simulink model "uncontrolled"  (R2020b)
settings: Solver=ode15s  StartTime=0  StopTime=5792.3373  MaxStep=0.1  RelTol=1e-8  AbsTol=1e-8
values from neighbouring files (symbols this model uses):
  data = struct()    [config.m]    (also in config6U.m; configSlew.m; mainOffNominal.m = dataFix)
libraries: simulink_extras x1
settings Model: SimulationMode=accelerator  Creator=pacif  LastModifiedBy=pacif

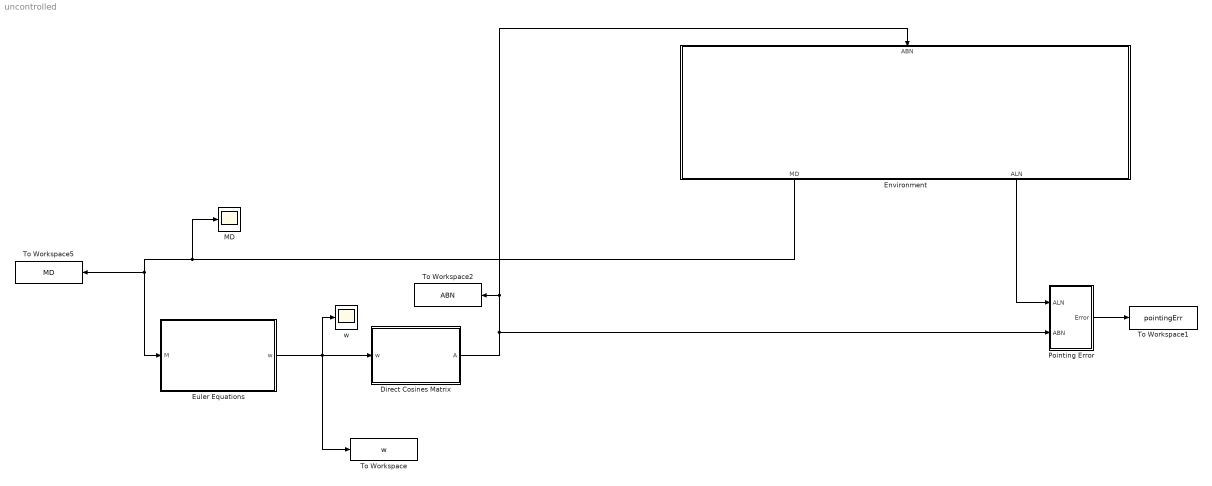
== system uncontrolled ==
  Direct Cosines Matrix : Subsystem
  Environment : Subsystem
  Euler Equations : Subsystem
  MD : Scope
  Pointing Error : Subsystem
  To Workspace : ToWorkspace  VariableName=w  SaveFormat=Timeseries  SampleTime=-1
  To Workspace1 : ToWorkspace  VariableName=pointingErr  SaveFormat=Timeseries  SampleTime=-1
  To Workspace2 : ToWorkspace  VariableName=ABN  SaveFormat=Timeseries  SampleTime=-1
  To Workspace5 : ToWorkspace  VariableName=MD  SaveFormat=Timeseries  SampleTime=-1
  w : Scope
  wires:
  Environment/1(MD) -> MD/1, To Workspace5/1, Euler Equations/1(M)
  Euler Equations/1(w) -> To Workspace/1, Direct Cosines Matrix/1(w), w/1
  Direct Cosines Matrix/1(A) -> To Workspace2/1, Environment/1(ABN), Pointing Error/2(ABN)
  Environment/2(ALN) -> Pointing Error/1(ALN)
  Pointing Error/1(Error) -> To Workspace1/1

== system uncontrolled/Direct Cosines Matrix ==
  w : Inport
  Build 3x3 Matrix : Subsystem
  Constant1 : Constant  Value=0
  Demux1 : Demux  Outputs=3
  Gain{3,5..7} (4 alike) : Gain  Gain=-1
  Integrator : Integrator  InitialCondition=data.ic.dcm
  Orthonormalization : Subsystem
  Product : Product  Multiplication=Matrix(*)
  A : Outport
  wires:
  Demux1/1 -> Build 3x3 Matrix/6(A32), Gain7/1
  Gain5/1 -> Build 3x3 Matrix/4(A12)
  Demux1/3 -> Build 3x3 Matrix/2(A21), Gain5/1
  Product/1 -> Gain3/1
  Build 3x3 Matrix/1(A) -> Product/1  "[w]^"
  Gain6/1 -> Build 3x3 Matrix/3(A31)
  Demux1/2 -> Build 3x3 Matrix/7("A13 "), Gain6/1
  Gain7/1 -> Build 3x3 Matrix/8(A23)
  Orthonormalization/1(A) -> Product/2, A/1
  Gain3/1 -> Integrator/1  "dA/dt"
  w/1 -> Demux1/1
  Integrator/1 -> Orthonormalization/1(A0)  "A"
  Constant1/1 -> Build 3x3 Matrix/1(A11), Build 3x3 Matrix/9(A33), Build 3x3 Matrix/5(A22)

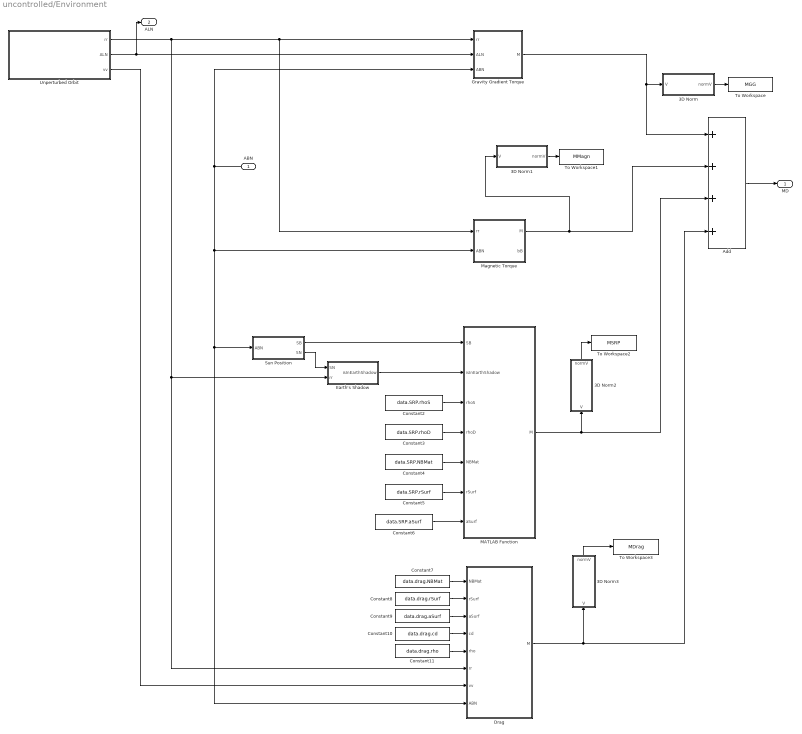
== system uncontrolled/Environment ==
  ABN : Inport
  3D Norm : Subsystem
  3D Norm1 : Subsystem
  3D Norm2 : Subsystem
  3D Norm3 : Subsystem
  Add : Sum  Inputs=++++
  Constant10 : Constant  Value=data.drag.cd
  Constant11 : Constant  Value=data.drag.rho
  Constant2 : Constant  Value=data.SRP.rhoS
  Constant3 : Constant  Value=data.SRP.rhoD
  Constant4 : Constant  Value=data.SRP.NBMat
  Constant5 : Constant  Value=data.SRP.rSurf
  Constant6 : Constant  Value=data.SRP.aSurf
  Constant7 : Constant  Value=data.drag.NBMat
  Constant8 : Constant  Value=data.drag.rSurf
  Constant9 : Constant  Value=data.drag.aSurf
  Drag : MATLAB Function  TreatAsAtomicUnit=on
  Earth's Shadow : Subsystem
  Gravity Gradient Torque : Subsystem
  MATLAB Function : MATLAB Function  TreatAsAtomicUnit=on
  Magnetic Torque : Subsystem
  "Sun Position " : Subsystem
  To Workspace : ToWorkspace  VariableName=MGG  SaveFormat=Timeseries  SampleTime=-1
  To Workspace1 : ToWorkspace  VariableName=MMagn  SaveFormat=Timeseries  SampleTime=-1
  To Workspace2 : ToWorkspace  VariableName=MSRP  SaveFormat=Timeseries  SampleTime=-1
  To Workspace3 : ToWorkspace  VariableName=MDrag  SaveFormat=Timeseries  SampleTime=-1
  Unperturbed Orbit : Subsystem
  MD : Outport
  ALN : Outport  Port=2
  wires:
  Earth's Shadow/1(isInEarthShadow) -> MATLAB Function/2(isInEarthShadow)
  Constant5/1 -> MATLAB Function/6(rSurf)
  Constant6/1 -> MATLAB Function/7(aSurf)
  Constant3/1 -> MATLAB Function/4(rhoD)
  Constant4/1 -> MATLAB Function/5(NBMat)
  Gravity Gradient Torque/1(M) -> 3D Norm/1(V), Add/1
  Unperturbed Orbit/1(rr) -> Earth's Shadow/2(rr), Drag/6(rr), Magnetic Torque/1(rr), Gravity Gradient Torque/1(rr)
  Constant10/1 -> Drag/4(cd)
  Drag/1(M) -> Add/4, 3D Norm3/1(V)
  ABN/1 -> Gravity Gradient Torque/3(ABN), Magnetic Torque/2(ABN), Drag/8(ABN), "Sun Position "/1(ABN)
  Constant7/1 -> Drag/1(NBMat)
  Constant8/1 -> Drag/2(rSurf)
  Constant9/1 -> Drag/3(aSurf)
  Add/1 -> MD/1
  Constant2/1 -> MATLAB Function/3(rhoS)
  Magnetic Torque/1(M) -> 3D Norm1/1(V), Add/2
  Unperturbed Orbit/2(ALN) -> ALN/1, Gravity Gradient Torque/2(ALN)
  Constant11/1 -> Drag/5(rho)
  Unperturbed Orbit/3(vv) -> Drag/7(vv)
  "Sun Position "/2(SN) -> Earth's Shadow/1(SN)
  "Sun Position "/1(SB) -> MATLAB Function/1(SB)
  MATLAB Function/1(M) -> Add/3, 3D Norm2/1(V)
  3D Norm/1(normV) -> To Workspace/1
  3D Norm1/1(normV) -> To Workspace1/1
  3D Norm2/1(normV) -> To Workspace2/1
  3D Norm3/1(normV) -> To Workspace3/1

== system uncontrolled/Euler Equations ==
  M : Inport
  Add : Sum
  Cross Product : Subsystem
  Gain : Gain  Gain=data.sc.invI  Multiplication=Matrix(K*u) (u vector)
  Gain2 : Gain  Gain=data.sc.inertiaMatrix  Multiplication=Matrix(K*u) (u vector)
  Integrator : Integrator  InitialCondition=data.ic.w
  w : Outport
  wires:
  Gain2/1 -> Cross Product/1(a)  "I*w"
  Cross Product/1(c) -> Add/2  "I*w x w = -w x I*w"
  M/1 -> Add/1
  Integrator/1 -> Cross Product/2(b), Gain2/1, w/1  "w"
  Gain/1 -> Integrator/1  "dw"
  Add/1 -> Gain/1

== system uncontrolled/Pointing Error ==
  ALN : Inport
  ABN : Inport  Port=2
  Acos : Trigonometry  Operator=acos
  Product : Product  Multiplication=Matrix(*)
  Radians to Degrees : simulink_extras/Transformations/Radians to Degrees
  Selector : Selector  NumberOfDimensions=2  InputPortWidth=3  IndexOptions=Index vector (dialog),Index vector (dialog)  Indices=1,1  OutputSizes=1,1
  Transpose : Math  Operator=transpose  SaturateOnIntegerOverflow=on
  Error : Outport
  wires:
  Radians to Degrees/1 -> Error/1
  ABN/1 -> Product/1
  ALN/1 -> Transpose/1
  Transpose/1 -> Product/2
  Product/1 -> Selector/1
  Selector/1 -> Acos/1
  Acos/1 -> Radians to Degrees/1

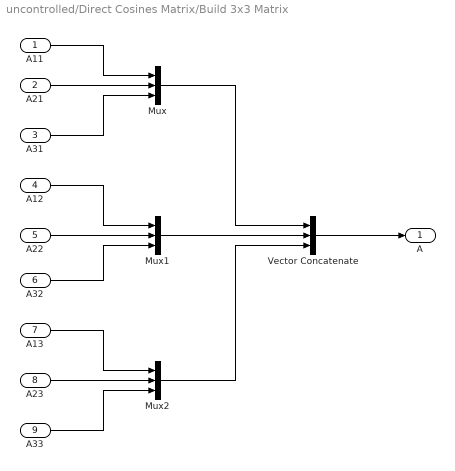
== system uncontrolled/Direct Cosines Matrix/Build 3x3 Matrix ==
  A11 : Inport
  A21 : Inport  Port=2
  A31 : Inport  Port=3
  A12 : Inport  Port=4
  A22 : Inport  Port=5
  A32 : Inport  Port=6
  "A13 " : Inport  Port=7
  A23 : Inport  Port=8
  A33 : Inport  Port=9
  Mux : Mux  Inputs=3
  Mux1 : Mux  Inputs=3
  Mux2 : Mux  Inputs=3
  Vector Concatenate : Concatenate  NumInputs=3  Mode=Multidimensional array  ConcatenateDimension=2
  A : Outport
  wires:
  A21/1 -> Mux/2
  A23/1 -> Mux2/2
  "A13 "/1 -> Mux2/1
  A11/1 -> Mux/1
  Vector Concatenate/1 -> A/1
  A31/1 -> Mux/3
  A12/1 -> Mux1/1
  A22/1 -> Mux1/2
  Mux2/1 -> Vector Concatenate/3
  Mux1/1 -> Vector Concatenate/2
  Mux/1 -> Vector Concatenate/1
  A33/1 -> Mux2/3
  A32/1 -> Mux1/3

== system uncontrolled/Direct Cosines Matrix/Orthonormalization ==
  A0 : Inport
  Add : Sum  Inputs=+-
  Gain : Gain  Gain=1.5
  Gain1 : Gain  Gain=0.5
  Product : Product  Inputs=3  Multiplication=Matrix(*)
  Transpose : Math  Operator=transpose  SaturateOnIntegerOverflow=on
  A : Outport
  wires:
  Add/1 -> A/1
  A0/1 -> Product/3, Transpose/1, Product/1, Gain/1
  Gain1/1 -> Add/2
  Gain/1 -> Add/1
  Transpose/1 -> Product/2
  Product/1 -> Gain1/1

== system uncontrolled/Environment/3D Norm ==
  V : Inport
  Add : Sum  Inputs=+++
  Demux : Demux  Outputs=3
  Square : Math  Operator=square  SaturateOnIntegerOverflow=on
  Square Root : Sqrt  SaturateOnIntegerOverflow=on
  Square1 : Math  Operator=square  SaturateOnIntegerOverflow=on
  Square2 : Math  Operator=square  SaturateOnIntegerOverflow=on
  normV : Outport
  wires:
  Square Root/1 -> normV/1
  V/1 -> Demux/1
  Demux/3 -> Square2/1
  Square/1 -> Add/1
  Demux/1 -> Square/1
  Demux/2 -> Square1/1
  Square2/1 -> Add/3
  Square1/1 -> Add/2
  Add/1 -> Square Root/1

== system uncontrolled/Environment/3D Norm1 ==
  V : Inport
  Add : Sum  Inputs=+++
  Demux : Demux  Outputs=3
  Square : Math  Operator=square  SaturateOnIntegerOverflow=on
  Square Root : Sqrt  SaturateOnIntegerOverflow=on
  Square1 : Math  Operator=square  SaturateOnIntegerOverflow=on
  Square2 : Math  Operator=square  SaturateOnIntegerOverflow=on
  normV : Outport
  wires:
  Square Root/1 -> normV/1
  V/1 -> Demux/1
  Demux/3 -> Square2/1
  Square/1 -> Add/1
  Demux/1 -> Square/1
  Demux/2 -> Square1/1
  Square2/1 -> Add/3
  Square1/1 -> Add/2
  Add/1 -> Square Root/1

== system uncontrolled/Environment/3D Norm2 ==
  V : Inport
  Add : Sum  Inputs=+++
  Demux : Demux  Outputs=3
  Square : Math  Operator=square  SaturateOnIntegerOverflow=on
  Square Root : Sqrt  SaturateOnIntegerOverflow=on
  Square1 : Math  Operator=square  SaturateOnIntegerOverflow=on
  Square2 : Math  Operator=square  SaturateOnIntegerOverflow=on
  normV : Outport
  wires:
  Square Root/1 -> normV/1
  V/1 -> Demux/1
  Demux/3 -> Square2/1
  Square/1 -> Add/1
  Demux/1 -> Square/1
  Demux/2 -> Square1/1
  Square2/1 -> Add/3
  Square1/1 -> Add/2
  Add/1 -> Square Root/1

== system uncontrolled/Environment/3D Norm3 ==
  V : Inport
  Add : Sum  Inputs=+++
  Demux : Demux  Outputs=3
  Square : Math  Operator=square  SaturateOnIntegerOverflow=on
  Square Root : Sqrt  SaturateOnIntegerOverflow=on
  Square1 : Math  Operator=square  SaturateOnIntegerOverflow=on
  Square2 : Math  Operator=square  SaturateOnIntegerOverflow=on
  normV : Outport
  wires:
  Square Root/1 -> normV/1
  V/1 -> Demux/1
  Demux/3 -> Square2/1
  Square/1 -> Add/1
  Demux/1 -> Square/1
  Demux/2 -> Square1/1
  Square2/1 -> Add/3
  Square1/1 -> Add/2
  Add/1 -> Square Root/1

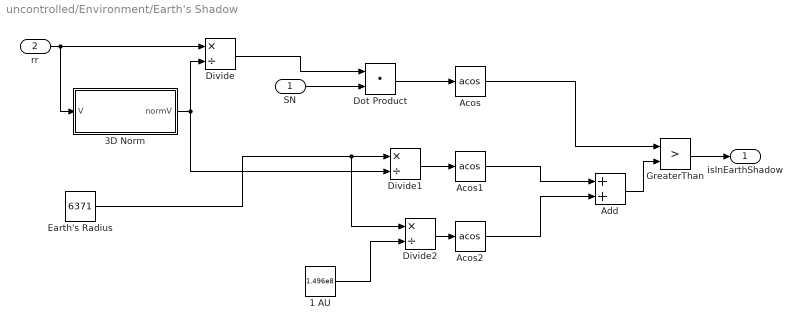
== system uncontrolled/Environment/Earth's Shadow ==
  SN : Inport
  rr : Inport  Port=2
  1 AU : Constant  Value=1.496e8
  3D Norm : Subsystem
  Acos : Trigonometry  Operator=acos
  Acos1 : Trigonometry  Operator=acos
  Acos2 : Trigonometry  Operator=acos
  Add : Sum
  Divide : Product  Inputs=*/
  Divide1 : Product  Inputs=*/
  Divide2 : Product  Inputs=*/
  Dot Product : DotProduct  InputSameDT=on  OutDataTypeStr=Inherit: Inherit via internal rule
  Earth's Radius : Constant  Value=6371
  GreaterThan : RelationalOperator  Operator=>  OutDataTypeStr=boolean  RndMeth=Simplest
  isInEarthShadow : Outport
  wires:
  SN/1 -> Dot Product/2
  GreaterThan/1 -> isInEarthShadow/1
  Add/1 -> GreaterThan/2
  Acos/1 -> GreaterThan/1
  Acos2/1 -> Add/2
  Acos1/1 -> Add/1
  rr/1 -> 3D Norm/1(V), Divide/1
  3D Norm/1(normV) -> Divide1/2, Divide/2
  Divide/1 -> Dot Product/1
  Dot Product/1 -> Acos/1
  Earth's Radius/1 -> Divide1/1, Divide2/1
  Divide1/1 -> Acos1/1
  Divide2/1 -> Acos2/1
  1 AU/1 -> Divide2/2

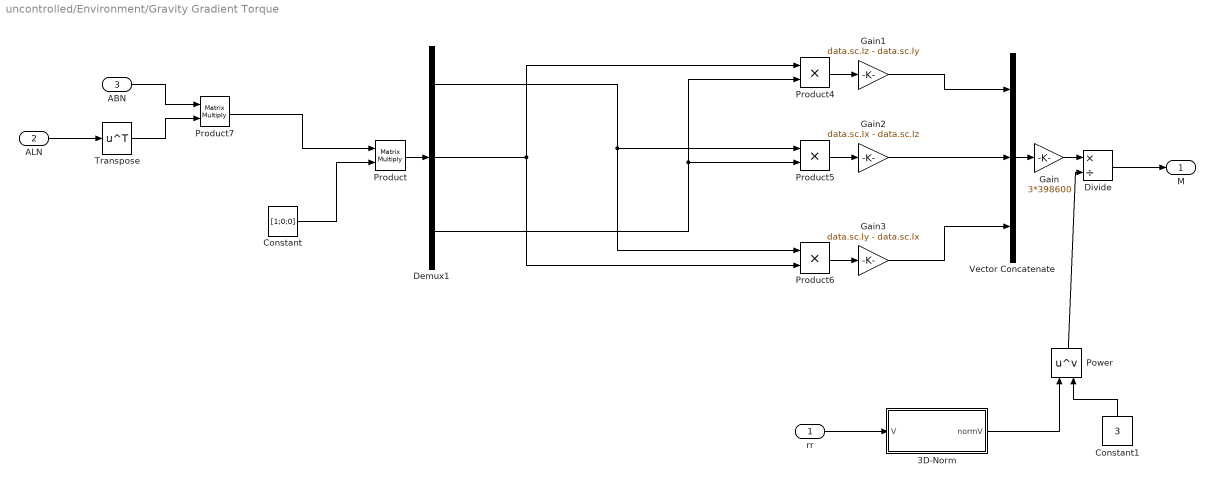
== system uncontrolled/Environment/Gravity Gradient Torque ==
  rr : Inport
  ALN : Inport  Port=2
  ABN : Inport  Port=3
  3D-Norm : Subsystem
  Constant : Constant  Value=[1;0;0]  VectorParams1D=off
  Constant1 : Constant  Value=3
  Demux1 : Demux  Outputs=3
  Divide : Product  Inputs=*/
  Gain : Gain  Gain=3*398600
  Gain1 : Gain  Gain=data.sc.Iz - data.sc.Iy
  Gain2 : Gain  Gain=data.sc.Ix - data.sc.Iz
  Gain3 : Gain  Gain=data.sc.Iy - data.sc.Ix
  Power : Math  Operator=pow  SaturateOnIntegerOverflow=on
  Product : Product  Multiplication=Matrix(*)
  Product4 : Product
  Product5 : Product
  Product6 : Product
  Product7 : Product  Multiplication=Matrix(*)
  Transpose : Math  Operator=transpose  SaturateOnIntegerOverflow=on
  Vector Concatenate : Concatenate  NumInputs=3
  M : Outport
  wires:
  Constant/1 -> Product/2
  Gain3/1 -> Vector Concatenate/3
  Gain1/1 -> Vector Concatenate/1
  Gain2/1 -> Vector Concatenate/2
  Vector Concatenate/1 -> Gain/1
  Constant1/1 -> Power/2
  Power/1 -> Divide/2
  Gain/1 -> Divide/1
  Product/1 -> Demux1/1
  Product4/1 -> Gain1/1
  Product5/1 -> Gain2/1
  Product6/1 -> Gain3/1
  Demux1/1 -> Product6/1, Product5/1
  Demux1/2 -> Product6/2, Product4/1
  Demux1/3 -> Product5/2, Product4/2
  Divide/1 -> M/1
  rr/1 -> 3D-Norm/1(V)
  3D-Norm/1(normV) -> Power/1
  ALN/1 -> Transpose/1
  Product7/1 -> Product/1
  ABN/1 -> Product7/1
  Transpose/1 -> Product7/2

== system uncontrolled/Environment/Magnetic Torque ==
  rr : Inport
  ABN : Inport  Port=2
  Cross Product : Subsystem
  Product : Product  Multiplication=Matrix(*)
  Subsystem : Subsystem
  m : Constant  Value=data.magneticTorque.m
  M : Outport
  bB : Outport  Port=2
  wires:
  rr/1 -> Subsystem/1(rr)
  ABN/1 -> Product/1
  Subsystem/1(bN) -> Product/2
  m/1 -> Cross Product/1(a)
  Product/1 -> Cross Product/2(b), bB/1
  Cross Product/1(c) -> M/1

== system uncontrolled/Environment/Sun Position  ==
  ABN : Inport
  Clock : Clock
  Cos : Trigonometry  Operator=cos
  Gain1 : Gain  Gain=2*pi/365/24/3600
  Gain2 : Gain  Gain=cos(23.45*pi/180)
  Gain3 : Gain  Gain=sin(23.45*pi/180)
  Mux : Mux  Inputs=3
  Product : Product  Multiplication=Matrix(*)
  Sin : Trigonometry
  Sin1 : Trigonometry
  SB : Outport
  SN : Outport  Port=2
  wires:
  Clock/1 -> Gain1/1
  Mux/1 -> SN/1, Product/2  "SN"
  Gain2/1 -> Mux/2
  Gain3/1 -> Mux/3
  Cos/1 -> Mux/1
  Sin1/1 -> Gain3/1
  Sin/1 -> Gain2/1
  Gain1/1 -> Sin/1, Sin1/1, Cos/1
  ABN/1 -> Product/1
  Product/1 -> SB/1

== system uncontrolled/Environment/Unperturbed Orbit ==
  Integrator : Integrator  InitialCondition=data.ic.th
  Subsystem : Subsystem
  Subsystem1 : Subsystem
  Subsystem2 : Subsystem
  Subsystem3 : Subsystem
  To Workspace : ToWorkspace  VariableName=theta  SaveFormat=Timeseries  SampleTime=-1
  rr : Outport
  ALN : Outport  Port=2
  vv : Outport  Port=3
  wires:
  Integrator/1 -> Subsystem2/1(theta), Subsystem1/1(theta), Subsystem3/1(theta), To Workspace/1, Subsystem/1(theta)
  Subsystem1/1(ALN) -> ALN/1
  Subsystem2/1(rr) -> rr/1
  Subsystem3/1(vv) -> vv/1
  Subsystem/1(theta_dot) -> Integrator/1

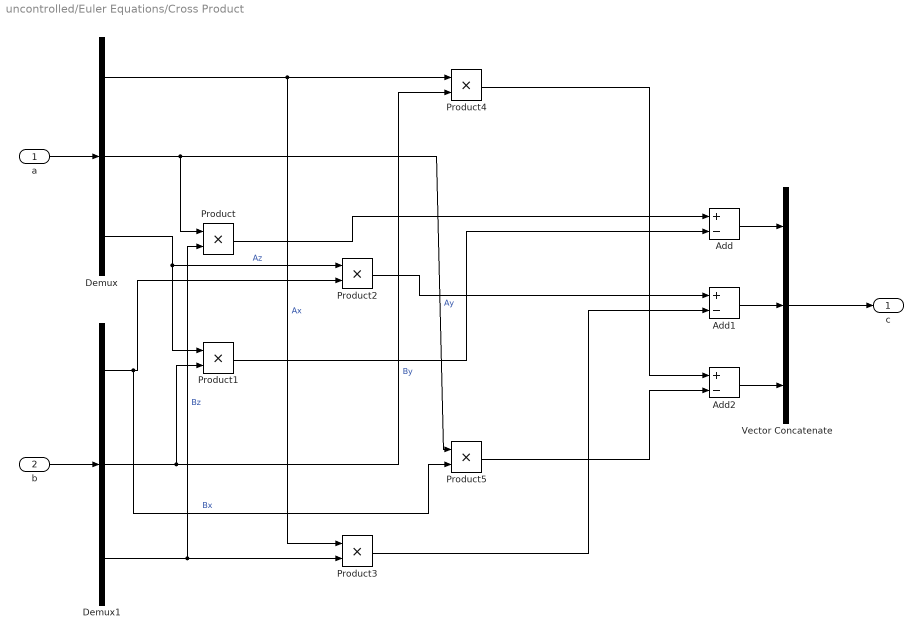
== system uncontrolled/Euler Equations/Cross Product ==
  a : Inport
  b : Inport  Port=2
  Add : Sum  Inputs=+-
  Add1 : Sum  Inputs=+-
  Add2 : Sum  Inputs=+-
  Demux : Demux  Outputs=3
  Demux1 : Demux  Outputs=3
  Product{,1..5} (6 alike) : Product
  Vector Concatenate : Concatenate  NumInputs=3
  c : Outport
  wires:
  Demux1/1 -> Product2/2, Product5/2  "Bx"
  Product2/1 -> Add1/1
  Vector Concatenate/1 -> c/1
  Add/1 -> Vector Concatenate/1
  Product3/1 -> Add1/2
  Product1/1 -> Add/2
  Product4/1 -> Add2/1
  Product/1 -> Add/1
  Demux/1 -> Product3/1, Product4/1  "Ax"
  Product5/1 -> Add2/2
  Demux/3 -> Product2/1, Product1/1  "Az"
  b/1 -> Demux1/1
  a/1 -> Demux/1
  Add2/1 -> Vector Concatenate/3
  Demux/2 -> Product5/1, Product/1  "Ay"
  Demux1/3 -> Product/2, Product3/2  "Bz"
  Demux1/2 -> Product4/2, Product1/2  "By"
  Add1/1 -> Vector Concatenate/2

== system uncontrolled/Environment/Earth's Shadow/3D Norm ==
  V : Inport
  Add : Sum  Inputs=+++
  Demux : Demux  Outputs=3
  Square : Math  Operator=square  SaturateOnIntegerOverflow=on
  Square Root : Sqrt  SaturateOnIntegerOverflow=on
  Square1 : Math  Operator=square  SaturateOnIntegerOverflow=on
  Square2 : Math  Operator=square  SaturateOnIntegerOverflow=on
  normV : Outport
  wires:
  Square Root/1 -> normV/1
  V/1 -> Demux/1
  Demux/3 -> Square2/1
  Square/1 -> Add/1
  Demux/1 -> Square/1
  Demux/2 -> Square1/1
  Square2/1 -> Add/3
  Square1/1 -> Add/2
  Add/1 -> Square Root/1

== system uncontrolled/Environment/Gravity Gradient Torque/3D-Norm ==
  V : Inport
  Add : Sum  Inputs=+++
  Demux : Demux  Outputs=3
  Square : Math  Operator=square  SaturateOnIntegerOverflow=on
  Square Root : Sqrt  SaturateOnIntegerOverflow=on
  Square1 : Math  Operator=square  SaturateOnIntegerOverflow=on
  Square2 : Math  Operator=square  SaturateOnIntegerOverflow=on
  normV : Outport
  wires:
  Square Root/1 -> normV/1
  Add/1 -> Square Root/1
  Square2/1 -> Add/3
  Square1/1 -> Add/2
  Square/1 -> Add/1
  Demux/1 -> Square/1
  Demux/2 -> Square1/1
  Demux/3 -> Square2/1
  V/1 -> Demux/1

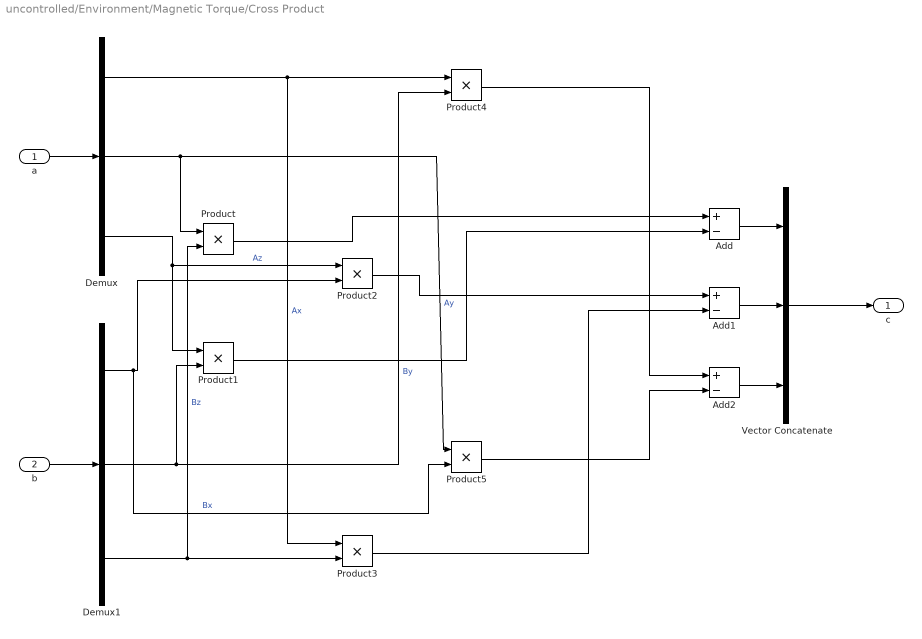
== system uncontrolled/Environment/Magnetic Torque/Cross Product ==
  a : Inport
  b : Inport  Port=2
  Add : Sum  Inputs=+-
  Add1 : Sum  Inputs=+-
  Add2 : Sum  Inputs=+-
  Demux : Demux  Outputs=3
  Demux1 : Demux  Outputs=3
  Product{,1..5} (6 alike) : Product
  Vector Concatenate : Concatenate  NumInputs=3
  c : Outport
  wires:
  Demux1/1 -> Product2/2, Product5/2  "Bx"
  Product2/1 -> Add1/1
  Vector Concatenate/1 -> c/1
  Add/1 -> Vector Concatenate/1
  Product3/1 -> Add1/2
  Product1/1 -> Add/2
  Product4/1 -> Add2/1
  Product/1 -> Add/1
  Demux/1 -> Product3/1, Product4/1  "Ax"
  Product5/1 -> Add2/2
  Demux/3 -> Product2/1, Product1/1  "Az"
  b/1 -> Demux1/1
  a/1 -> Demux/1
  Add2/1 -> Vector Concatenate/3
  Demux/2 -> Product5/1, Product/1  "Ay"
  Demux1/3 -> Product/2, Product3/2  "Bz"
  Demux1/2 -> Product4/2, Product1/2  "By"
  Add1/1 -> Vector Concatenate/2

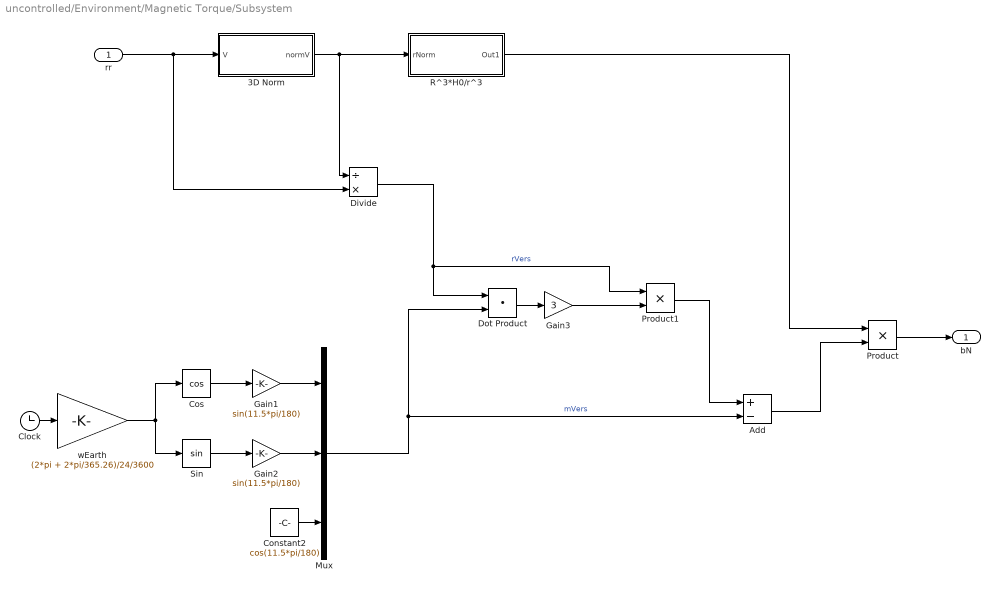
== system uncontrolled/Environment/Magnetic Torque/Subsystem ==
  rr : Inport
  3D Norm : Subsystem
  Add : Sum  Inputs=+-
  Clock : Clock
  Constant2 : Constant  Value=cos(11.5*pi/180)
  Cos : Trigonometry  Operator=cos
  Divide : Product  Inputs=/*
  Dot Product : DotProduct  InputSameDT=on  OutDataTypeStr=Inherit: Inherit via internal rule
  Gain1 : Gain  Gain=sin(11.5*pi/180)
  Gain2 : Gain  Gain=sin(11.5*pi/180)
  Gain3 : Gain  Gain=3
  Mux : Mux  Inputs=3
  Product : Product
  Product1 : Product
  R^3*H0/r^3 : Subsystem
  Sin : Trigonometry
  wEarth : Gain  Gain=(2*pi + 2*pi/365.26)/24/3600
  bN : Outport
  wires:
  3D Norm/1(normV) -> Divide/1, R^3*H0/r^3/1(rNorm)
  Cos/1 -> Gain1/1
  Sin/1 -> Gain2/1
  Gain2/1 -> Mux/2
  rr/1 -> 3D Norm/1(V), Divide/2
  Product1/1 -> Add/1
  wEarth/1 -> Sin/1, Cos/1
  Constant2/1 -> Mux/3
  Gain1/1 -> Mux/1
  Gain3/1 -> Product1/2
  Product/1 -> bN/1
  Add/1 -> Product/2
  Clock/1 -> wEarth/1
  R^3*H0/r^3/1(Out1) -> Product/1
  Dot Product/1 -> Gain3/1
  Divide/1 -> Product1/1, Dot Product/1  "rVers"
  Mux/1 -> Dot Product/2, Add/2  "mVers"

== system uncontrolled/Environment/Unperturbed Orbit/Subsystem ==
  theta : Inport
  Add : Sum
  Constant : Constant
  Cos : Trigonometry  Operator=cos
  Gain : Gain  Gain=data.orbit.e
  Gain1 : Gain  Gain=data.orbit.n/(1-data.orbit.e^2)^(3/2)
  Square : Math  Operator=square  SaturateOnIntegerOverflow=on
  theta_dot : Outport
  wires:
  theta/1 -> Cos/1
  Cos/1 -> Gain/1
  Gain/1 -> Add/1
  Constant/1 -> Add/2
  Add/1 -> Square/1
  Square/1 -> Gain1/1
  Gain1/1 -> theta_dot/1

== system uncontrolled/Environment/Unperturbed Orbit/Subsystem1 ==
  theta : Inport
  Build 3x3 Matrix : Subsystem
  Constant : Constant  Value=0
  Constant1 : Constant
  Cos1 : Trigonometry  Operator=cos
  Cos2 : Trigonometry  Operator=cos
  Gain : Gain  Gain=-1
  Gain1 : Gain  Gain=[1 0 0; 0 cos(data.orbit.i) sin(data.orbit.i); 0 -sin(data.orbit.i) cos(data.orbit.i)]  Multiplication=Matrix(u*K)
  Sin : Trigonometry
  Sin1 : Trigonometry
  ALN : Outport
  wires:
  Cos1/1 -> Build 3x3 Matrix/1(A11)
  theta/1 -> Cos2/1, Sin1/1, Cos1/1, Sin/1
  Sin/1 -> Gain/1
  Gain/1 -> Build 3x3 Matrix/2(A21)
  Sin1/1 -> Build 3x3 Matrix/4(A12)
  Cos2/1 -> Build 3x3 Matrix/5(A22)
  Constant/1 -> Build 3x3 Matrix/8(A23), Build 3x3 Matrix/7("A13 "), Build 3x3 Matrix/6(A32), Build 3x3 Matrix/3(A31)
  Constant1/1 -> Build 3x3 Matrix/9(A33)
  Build 3x3 Matrix/1(A) -> Gain1/1
  Gain1/1 -> ALN/1

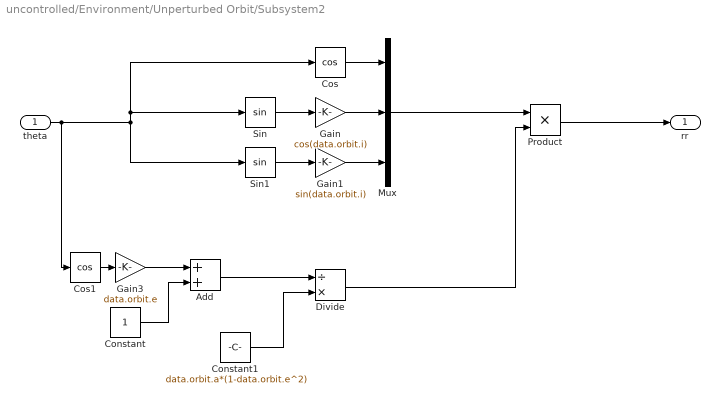
== system uncontrolled/Environment/Unperturbed Orbit/Subsystem2 ==
  theta : Inport
  Add : Sum
  Constant : Constant
  Constant1 : Constant  Value=data.orbit.a*(1-data.orbit.e^2)
  Cos : Trigonometry  Operator=cos
  Cos1 : Trigonometry  Operator=cos
  Divide : Product  Inputs=/*
  Gain : Gain  Gain=cos(data.orbit.i)
  Gain1 : Gain  Gain=sin(data.orbit.i)
  Gain3 : Gain  Gain=data.orbit.e
  Mux : Mux  Inputs=3
  Product : Product
  Sin : Trigonometry
  Sin1 : Trigonometry
  rr : Outport
  wires:
  Cos/1 -> Mux/1
  theta/1 -> Cos1/1, Sin1/1, Cos/1, Sin/1
  Gain/1 -> Mux/2
  Gain1/1 -> Mux/3
  Sin/1 -> Gain/1
  Sin1/1 -> Gain1/1
  Cos1/1 -> Gain3/1
  Gain3/1 -> Add/1
  Constant/1 -> Add/2
  Add/1 -> Divide/1
  Constant1/1 -> Divide/2
  Divide/1 -> Product/2
  Mux/1 -> Product/1
  Product/1 -> rr/1

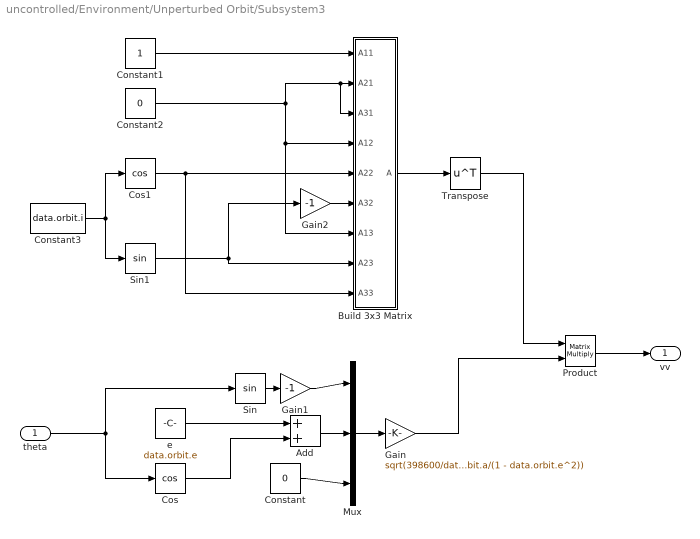
== system uncontrolled/Environment/Unperturbed Orbit/Subsystem3 ==
  theta : Inport
  Add : Sum
  Build 3x3 Matrix : Subsystem
  Constant : Constant  Value=0
  Constant1 : Constant
  Constant2 : Constant  Value=0
  Constant3 : Constant  Value=data.orbit.i
  Cos : Trigonometry  Operator=cos
  Cos1 : Trigonometry  Operator=cos
  Gain : Gain  Gain=sqrt(398600/data.orbit.a/(1 - data.orbit.e^2))
  Gain1 : Gain  Gain=-1
  Gain2 : Gain  Gain=-1
  Mux : Mux  Inputs=3
  Product : Product  Multiplication=Matrix(*)
  Sin : Trigonometry
  Sin1 : Trigonometry
  Transpose : Math  Operator=transpose  SaturateOnIntegerOverflow=on
  e : Constant  Value=data.orbit.e
  vv : Outport
  wires:
  Mux/1 -> Gain/1
  theta/1 -> Cos/1, Sin/1
  Constant/1 -> Mux/3
  Add/1 -> Mux/2
  Cos/1 -> Add/2
  Sin/1 -> Gain1/1
  e/1 -> Add/1
  Gain1/1 -> Mux/1
  Constant3/1 -> Sin1/1, Cos1/1
  Constant1/1 -> Build 3x3 Matrix/1(A11)
  Constant2/1 -> Build 3x3 Matrix/3(A31), Build 3x3 Matrix/2(A21), Build 3x3 Matrix/4(A12), Build 3x3 Matrix/7("A13 ")
  Cos1/1 -> Build 3x3 Matrix/9(A33), Build 3x3 Matrix/5(A22)
  Gain2/1 -> Build 3x3 Matrix/6(A32)
  Sin1/1 -> Build 3x3 Matrix/8(A23), Gain2/1
  Build 3x3 Matrix/1(A) -> Transpose/1
  Transpose/1 -> Product/1
  Gain/1 -> Product/2
  Product/1 -> vv/1

== system uncontrolled/Environment/Magnetic Torque/Subsystem/3D Norm ==
  V : Inport
  Add : Sum  Inputs=+++
  Demux : Demux  Outputs=3
  Square : Math  Operator=square  SaturateOnIntegerOverflow=on
  Square Root : Sqrt  SaturateOnIntegerOverflow=on
  Square1 : Math  Operator=square  SaturateOnIntegerOverflow=on
  Square2 : Math  Operator=square  SaturateOnIntegerOverflow=on
  normV : Outport
  wires:
  Square Root/1 -> normV/1
  V/1 -> Demux/1
  Demux/3 -> Square2/1
  Square/1 -> Add/1
  Demux/1 -> Square/1
  Demux/2 -> Square1/1
  Square2/1 -> Add/3
  Square1/1 -> Add/2
  Add/1 -> Square Root/1

== system uncontrolled/Environment/Magnetic Torque/Subsystem/R^3*H0//r^3 ==
  rNorm : Inport
  Constant : Constant  Value=3
  Constant1 : Constant  Value=3
  Divide : Product  Inputs=**/
  H0 : Constant  Value=((-29615e-9)^2 + (-1728e-9)^2 + 5186e-9^2)^(1/2)
  Power : Math  Operator=pow  SaturateOnIntegerOverflow=on
  Power1 : Math  Operator=pow  SaturateOnIntegerOverflow=on
  R_EARTH : Constant  Value=6371
  Out1 : Outport
  wires:
  H0/1 -> Divide/2
  Power/1 -> Divide/1
  Power1/1 -> Divide/3
  Divide/1 -> Out1/1
  Constant1/1 -> Power1/2
  rNorm/1 -> Power1/1
  Constant/1 -> Power/2
  R_EARTH/1 -> Power/1

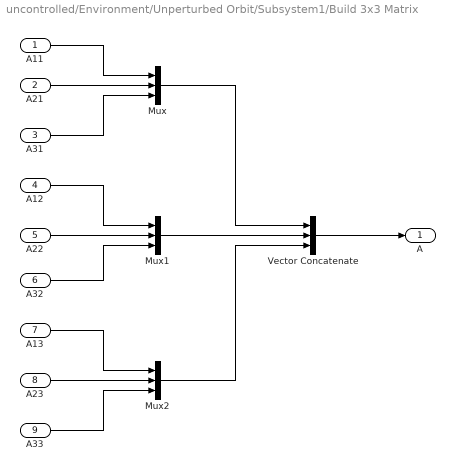
== system uncontrolled/Environment/Unperturbed Orbit/Subsystem1/Build 3x3 Matrix ==
  A11 : Inport
  A21 : Inport  Port=2
  A31 : Inport  Port=3
  A12 : Inport  Port=4
  A22 : Inport  Port=5
  A32 : Inport  Port=6
  "A13 " : Inport  Port=7
  A23 : Inport  Port=8
  A33 : Inport  Port=9
  Mux : Mux  Inputs=3
  Mux1 : Mux  Inputs=3
  Mux2 : Mux  Inputs=3
  Vector Concatenate : Concatenate  NumInputs=3  Mode=Multidimensional array  ConcatenateDimension=2
  A : Outport
  wires:
  A21/1 -> Mux/2
  A23/1 -> Mux2/2
  "A13 "/1 -> Mux2/1
  A11/1 -> Mux/1
  Vector Concatenate/1 -> A/1
  A31/1 -> Mux/3
  A12/1 -> Mux1/1
  A22/1 -> Mux1/2
  Mux2/1 -> Vector Concatenate/3
  Mux1/1 -> Vector Concatenate/2
  Mux/1 -> Vector Concatenate/1
  A33/1 -> Mux2/3
  A32/1 -> Mux1/3

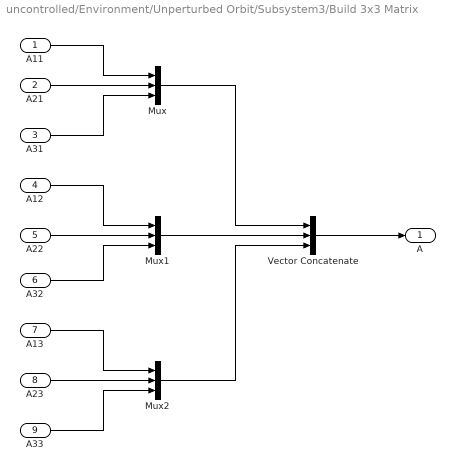
== system uncontrolled/Environment/Unperturbed Orbit/Subsystem3/Build 3x3 Matrix ==
  A11 : Inport
  A21 : Inport  Port=2
  A31 : Inport  Port=3
  A12 : Inport  Port=4
  A22 : Inport  Port=5
  A32 : Inport  Port=6
  "A13 " : Inport  Port=7
  A23 : Inport  Port=8
  A33 : Inport  Port=9
  Mux : Mux  Inputs=3
  Mux1 : Mux  Inputs=3
  Mux2 : Mux  Inputs=3
  Vector Concatenate : Concatenate  NumInputs=3  Mode=Multidimensional array  ConcatenateDimension=2
  A : Outport
  wires:
  A21/1 -> Mux/2
  A23/1 -> Mux2/2
  "A13 "/1 -> Mux2/1
  A11/1 -> Mux/1
  Vector Concatenate/1 -> A/1
  A31/1 -> Mux/3
  A12/1 -> Mux1/1
  A22/1 -> Mux1/2
  Mux2/1 -> Vector Concatenate/3
  Mux1/1 -> Vector Concatenate/2
  Mux/1 -> Vector Concatenate/1
  A33/1 -> Mux2/3
  A32/1 -> Mux1/3

== matlab function uncontrolled/Environment/Drag ==
  data: NBMat input; M output; rSurf input; aSurf input; cd input; rho input; rr input; vv input; ABN input
function M = fcn(NBMat,rSurf,aSurf,cd,rho,rr,vv,ABN)

wEarth = 0.000072921;

rr = rr*1e3; vv = vv*1e3;

vRel = ABN*[vv(1) + wEarth*rr(1); vv(2) - wEarth*rr(2); vv(3)];

nSurf = size(NBMat,2);

M = [0; 0; 0];

for i = 1:nSurf
    
    NBi = NBMat(:,i); ri = rSurf(:,i); Ai = aSurf(i);
    
    Ki = dot(vRel/norm(vRel),NBi); 
    
    if Ki > 0
        
        Fi = -0.5*rho*cd*norm(vRel)*vRel*Ai*Ki;
        
        M = M + cross(ri,Fi);
        
    end
    
end

end

== matlab function uncontrolled/Environment/MATLAB Function ==
  data: SB input; isInEarthShadow input; rhoS input; rhoD input; NBMat input; rSurf input; aSurf input; M output
function M = SRP(SB,isInEarthShadow,rhoS,rhoD,NBMat,rSurf,aSurf)

% Constants:
Fe = 1975; c = 3e8; P = Fe/c;

nSurf = size(NBMat,2);

M = [0; 0; 0];

if ~isInEarthShadow
    
    for i = 1:nSurf
        
        NBi = NBMat(:,i); ri = rSurf(:,i); Ai = aSurf(i);
        rhoSi = rhoS(i); rhoDi = rhoD(i);
        
        Ki = dot(SB,NBi);
        
        if Ki > 0
            
            Fi = -P*Ai*Ki*((1-rhoSi)*SB +...
                (2*rhoSi*Ki + 2/3*rhoDi)*NBi);
            
            M = M + cross(ri,Fi);
            
        end
        
    end
    
end
end
